simulink model "fuzzy_model"  (R2012b)
settings: Solver=ode45  StartTime=0.0  StopTime=20  RelTol=1e-3
libraries: fuzblock x4
settings Model: Creator=2Filipek  LastModifiedBy=Amadeusz

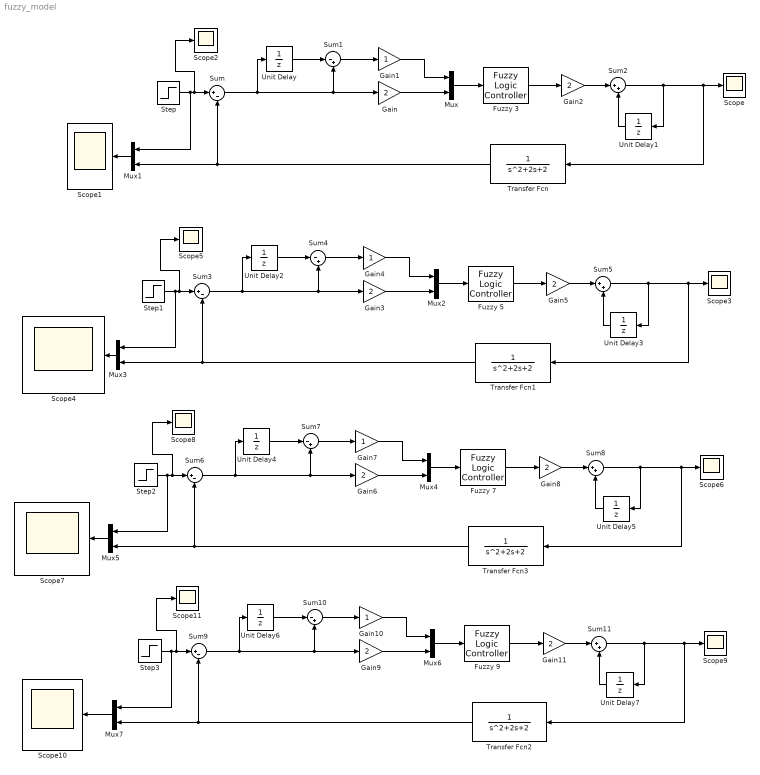
== system fuzzy_model ==
  Fuzzy 3 : fuzblock/Fuzzy Logic  Controller  fis=['fuzzy_3']
  Fuzzy 5 : fuzblock/Fuzzy Logic  Controller  fis=['fuzzy_5']
  Fuzzy 7 : fuzblock/Fuzzy Logic  Controller  fis=['fuzzy_7']
  Fuzzy 9 : fuzblock/Fuzzy Logic  Controller  fis=['fuzzy_9']
  Gain{,2..3,5..6,8..9,11} (8 alike) : Gain  Gain=2
  Gain{1,4,7,10} (4 alike) : Gain
  Mux{,1..7} (8 alike) : Mux  Inputs=2
  Scope{,1..11} (12 alike) : Scope
      Scope1 settings: TimeRange=2  YMin=-0.5030181086519105  YMax=0.3420523138833005
      Scope10 settings: TimeRange=2  YMin=-0.5030181086519105  YMax=0.3420523138833005  SaveName=ScopeData9
      Scope11 settings: SaveName=ScopeData10
      Scope2 settings: SaveName=ScopeData2
      Scope3 settings: SaveName=ScopeData3
      Scope4 settings: TimeRange=2  YMin=-0.5030181086519105  YMax=0.3420523138833005  SaveName=ScopeData4
      Scope5 settings: SaveName=ScopeData5
      Scope6 settings: SaveName=ScopeData6
      Scope7 settings: TimeRange=2  YMin=-0.5030181086519105  YMax=0.3420523138833005  SaveName=ScopeData7
      Scope8 settings: SaveName=ScopeData8
      Scope9 settings: SaveName=ScopeData11
  Step{,1..3} (4 alike) : Step  SampleTime=0
  Sum{,3,6,9} (4 alike) : Sum  Inputs=|+-
  Sum{1,4,7,10} (4 alike) : Sum  Inputs=|-+
  Sum{2,5,8,11} (4 alike) : Sum  Inputs=|++
  Transfer Fcn{,1..3} (4 alike) : TransferFcn  Denominator=[1 2 2]
  Unit Delay{,1..2,4,6} (5 alike) : UnitDelay
  Unit Delay3 : UnitDelay  InitialCondition=1
  Unit Delay5 : UnitDelay  InitialCondition=1
  Unit Delay7 : UnitDelay  InitialCondition=1
  wires:
  Mux/1 -> Fuzzy 3/1
  Sum/1 -> Unit Delay/1, Sum1/2, Gain/1
  Unit Delay/1 -> Sum1/1
  Gain/1 -> Mux/2
  Sum1/1 -> Gain1/1
  Gain1/1 -> Mux/1
  Fuzzy 3/1 -> Gain2/1
  Gain2/1 -> Sum2/1
  Unit Delay1/1 -> Sum2/2
  Sum2/1 -> Unit Delay1/1, Scope/1, Transfer Fcn/1
  Transfer Fcn/1 -> Mux1/2, Sum/2
  Step/1 -> Mux1/1, Scope2/1, Sum/1
  Mux1/1 -> Scope1/1
  Mux2/1 -> Fuzzy 5/1
  Sum3/1 -> Unit Delay2/1, Sum4/2, Gain3/1
  Unit Delay2/1 -> Sum4/1
  Gain3/1 -> Mux2/2
  Sum4/1 -> Gain4/1
  Gain4/1 -> Mux2/1
  Fuzzy 5/1 -> Gain5/1
  Gain5/1 -> Sum5/1
  Unit Delay3/1 -> Sum5/2
  Sum5/1 -> Unit Delay3/1, Scope3/1, Transfer Fcn1/1
  Transfer Fcn1/1 -> Mux3/2, Sum3/2
  Step1/1 -> Mux3/1, Scope5/1, Sum3/1
  Mux3/1 -> Scope4/1
  Mux4/1 -> Fuzzy 7/1
  Sum6/1 -> Unit Delay4/1, Sum7/2, Gain6/1
  Unit Delay4/1 -> Sum7/1
  Gain6/1 -> Mux4/2
  Sum7/1 -> Gain7/1
  Gain7/1 -> Mux4/1
  Fuzzy 7/1 -> Gain8/1
  Gain8/1 -> Sum8/1
  Unit Delay5/1 -> Sum8/2
  Sum8/1 -> Unit Delay5/1, Scope6/1, Transfer Fcn3/1
  Transfer Fcn3/1 -> Mux5/2, Sum6/2
  Step2/1 -> Mux5/1, Scope8/1, Sum6/1
  Mux5/1 -> Scope7/1
  Mux6/1 -> Fuzzy 9/1
  Sum9/1 -> Unit Delay6/1, Sum10/2, Gain9/1
  Unit Delay6/1 -> Sum10/1
  Gain9/1 -> Mux6/2
  Sum10/1 -> Gain10/1
  Gain10/1 -> Mux6/1
  Fuzzy 9/1 -> Gain11/1
  Gain11/1 -> Sum11/1
  Unit Delay7/1 -> Sum11/2
  Sum11/1 -> Unit Delay7/1, Scope9/1, Transfer Fcn2/1
  Transfer Fcn2/1 -> Mux7/2, Sum9/2
  Step3/1 -> Mux7/1, Scope11/1, Sum9/1
  Mux7/1 -> Scope10/1
